simulink model "gyro_read"  (R2020a)
settings: Solver=FixedStepDiscrete  StartTime=0.0  StopTime=10.0  RelTol=1e-3  EnableMultiTasking=on
undefined symbols (not defined in the file): ESP, IDF, IP, TCP
libraries: esp32_i2c_lib x15, simulink x5, waijung2_utilities_lib x4, esp32_device_config_lib x1
settings Model: Creator=Aimagin  LastModifiedBy=Aimagin
settings SolverCC: PositivePriorityOrder=on  AutoInsertRateTranBlk=on
settings OptimizationCC: DefaultParameterBehavior=Inlined  EnhancedBackFolding=on  PassReuseOutputArgsAs=Individual arguments  ZeroExternalMemoryAtStartup=off  ZeroInternalMemoryAtStartup=off  OptimizeBlockOrder=speed  DifferentSizesBufferReuse=on  OptimizationCustomize=off  EfficientTunableParamExpr=on
settings DebuggingCC: ParameterTunabilityLossMsg=error
settings HardwareCC: ProdBitPerPointer=32  ProdBitPerSizeT=32  ProdBitPerPtrDiffT=32  ProdLargestAtomicInteger=Long  ProdLargestAtomicFloat=Double  ProdWordSize=32  ProdHWDeviceType=Cadence Design Systems (Tensilica)->Espressif Xtensa single-/dual-core 32-bit LX6 microprocessor
settings SFSimCC: MATLABDynamicMemAlloc=off
settings RTWCC: Description=Waijung 2 ESP32 target  SystemTargetFile=esp32.tlc  TemplateMakefile=esp32.tmf  RetainRTWFile=on
settings CodeAppCC: ForceParamTrailComments=on  IgnoreCustomStorageClasses=off  OperatorAnnotations=on  SimulinkDataObjDesc=on  SFDataObjDesc=on  InsertBlockDesc=on
settings STFCustomTargetCC: TargetLangStandard=C99 (ISO)  MultiwordLength=256  ModelReferenceCompliant=off  CombineOutputUpdateFcns=on  ERTCustomFileBanners=on  SupportContinuousTime=off  SupportNonInlinedSFcns=off  RemoveResetFunc=on  MATLABClassNameForMDSCustomization=Simulink.SoftwareTarget.ERTCustomization  SystemTargetFile=esp32.tlc
settings ERTTargetCC: TargetLangStandard=C99 (ISO)  ModelReferenceCompliant=off  ParMdlRefBuildCompliant=off  CompOptLevelCompliant=off  ConcurrentExecutionCompliant=off  ModelStepFunctionPrototypeControlCompliant=off  CPPClassGenCompliant=off  UseToolchainInfoCompliant=off  ExtModeStaticAlloc=on  ExtModeStaticAllocSize=2048  InlinedParameterPlacement=NonHierarchical  ERTSrcFileBannerTemplate=esp32_code_template.cgt  ERTHdrFileBannerTemplate=esp32_code_template.cgt  ERTDataSrcFileTemplate=esp32_code_template.cgt  ERTDataHdrFileTemplate=esp32_code_template.cgt  ERTCustomFileTemplate=esp32_file_process.tlc

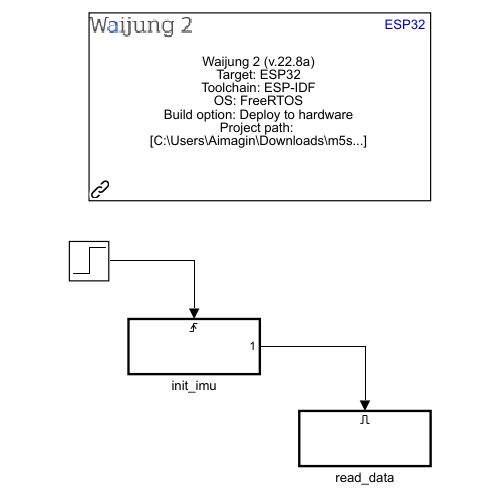
[thumbnail: Simulink's stored preview of the top-level diagram]
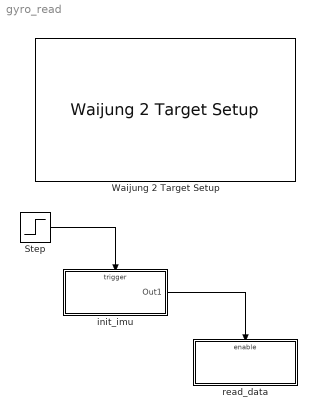
== system gyro_read ==
  Step : Step  SampleTime=0.2
  Waijung 2 Target Setup : esp32_device_config_lib/Waijung 2 Target Setup  waijungversion=22.8a  toolchain=ESP-IDF  os=FreeRTOS  sampletime=-1  simulink_managebuildsystem=on  projectpath=C:\Users\Aimagin\Downloads\m5stick_wrkshop\gyro_read_esp32_build_system  espidfpath=C:\msys32\home\skris\esp\esp-idf  buildoptions=Deploy to hardware  blockid=Waijung2TargetSetup  target=ESP32  defaultstacksize=2048  basepriority=0  highestpriority=10  generate_baserate_task=on  tickrate=1000  esp32target=ESP32  esp32targetdef=esp32  esp32flashsize=4MB  esp32comport=COM8  esp32baudrate=115200  esp32advancedconfig=off  esp32partitiontable=Use default waijung2 partition table  esp32partitionpath=Browse the partition table  partitionname=partitions.csv  editpartition=off  custompartitiondata={'nvs','data','nvs','','0x6000','';'phy_init','data','phy','','0x1000','';'factory','app','factory','','1M',''}  reqblocks=default  esp32custompartition={'nvs','data','nvs','','0x6000','';'phy_init','data','phy','','0x1000','';'factory','app','factory','','1M',''}  cominterface=TCP/IP  wifimode=WIFI AP  wifissid=esp32ssid  wifipassword=password  deviceip=192.168.1.10  targetgateway=192.168.1.1  targetnetmask=255.255.255.0  manualdns=on  targetdnsip=8.8.8.8  targetipport=256  targetipdef=0  targetmaskdef=0  targetgatewaydef=0  targetdnsipdef=0  hosttimeout=10  hostverbose=off
      settings: SourceProductName=Waijung 2 Blockset
  init_imu : Subsystem  TreatAsAtomicUnit=on
  read_data : Subsystem  TreatAsAtomicUnit=on
  wires:
  Step/1 -> init_imu/Trigger
  init_imu/1(Out1) -> read_data/Enable

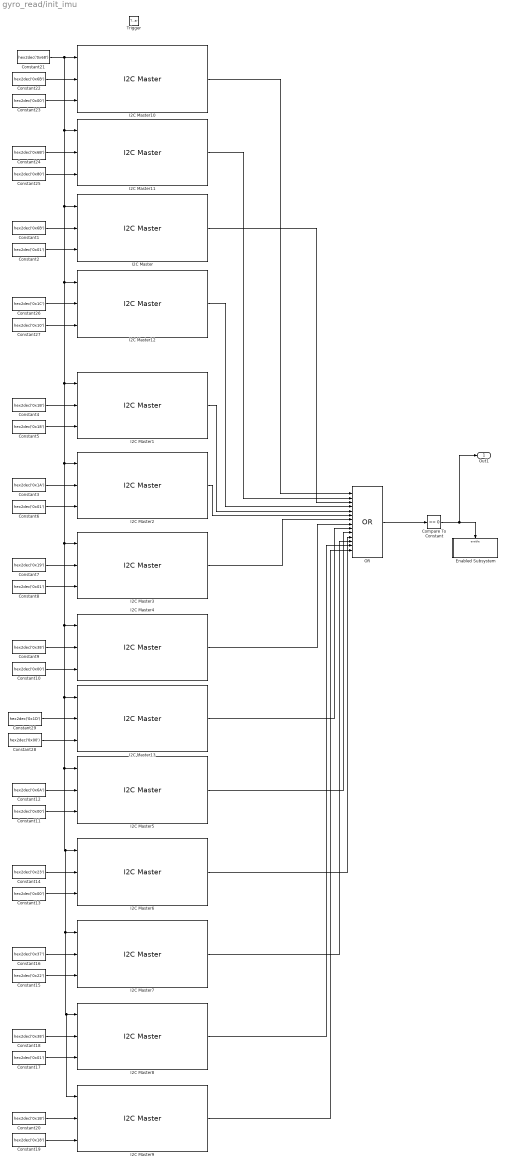
== system gyro_read/init_imu ==
  Trigger : TriggerPort  VariantControl=Variant
  Compare To Constant : simulink/Logic and Bit Operations/Compare To Constant  relop===  const=0  OutDataTypeStr=boolean
  Constant1 : Constant  Value=hex2dec('0x6B')  SampleTime=-1
  Constant{10..11,13,23,28} (5 alike) : Constant  Value=hex2dec('0x00')  SampleTime=-1
  Constant12 : Constant  Value=hex2dec('0x6A')  SampleTime=-1
  Constant14 : Constant  Value=hex2dec('0x23')  SampleTime=-1
  Constant15 : Constant  Value=hex2dec('0x22')  SampleTime=-1
  Constant16 : Constant  Value=hex2dec('0x37')  SampleTime=-1
  Constant{2,6,8,17} (4 alike) : Constant  Value=hex2dec('0x01')  SampleTime=-1
  Constant18 : Constant  Value=hex2dec('0x38')  SampleTime=-1
  Constant19 : Constant  Value=hex2dec('0x18')  SampleTime=-1
  Constant20 : Constant  Value=hex2dec('0x1B')  SampleTime=-1
  Constant21 : Constant  Value=hex2dec('0x68')  SampleTime=-1
  Constant22 : Constant  Value=hex2dec('0x6B')  SampleTime=-1
  Constant24 : Constant  Value=hex2dec('0x6B')  SampleTime=-1
  Constant25 : Constant  Value=hex2dec('0x80')  SampleTime=-1
  Constant26 : Constant  Value=hex2dec('0x1C')  SampleTime=-1
  Constant27 : Constant  Value=hex2dec('0x10')  SampleTime=-1
  Constant29 : Constant  Value=hex2dec('0x1D')  SampleTime=-1
  Constant3 : Constant  Value=hex2dec('0x1A')  SampleTime=-1
  Constant4 : Constant  Value=hex2dec('0x1B')  SampleTime=-1
  Constant5 : Constant  Value=hex2dec('0x18')  SampleTime=-1
  Constant7 : Constant  Value=hex2dec('0x19')  SampleTime=-1
  Constant9 : Constant  Value=hex2dec('0x38')  SampleTime=-1
  Enabled Subsystem : Subsystem  TreatAsAtomicUnit=on
  I2C Master : esp32_i2c_lib/I2C Master  blockid=init_imuI2CMaster  mode=Continuous  i2cinit=on  i2cport=0  i2cportdef=I2C_NUM_0  clkspeed=100  overridepin=off  sdapin=21  sdapinpull=Enable  sclpin=22  sclpinpull=Enable  inputcount=2  outputcount=0  enablelog=off  inputportlabel={'SlvAddr' 'Wr0 (uint8)' 'Wr1 (uint8)' }  outputportlabel={'Status' '(uint8) Rd0' '(uint8) Rd1' }  sdapinpulldef=GPIO_PULLUP_ENABLE  sclpinpulldef=GPIO_PULLUP_ENABLE  enablelogdef=0  sampletime=-1  sampletimestr=2
      settings: SourceProductName=Waijung 2 Blockset
  I2C Master1 : esp32_i2c_lib/I2C Master  blockid=init_imuI2CMaster1  mode=Continuous  i2cinit=off  i2cport=0  i2cportdef=I2C_NUM_0  clkspeed=100  overridepin=off  sdapin=21  sdapinpull=Enable  sclpin=22  sclpinpull=Enable  inputcount=2  outputcount=0  enablelog=off  inputportlabel={'SlvAddr' 'Wr0 (uint8)' 'Wr1 (uint8)' }  outputportlabel={'Status' '(uint8) Rd0' '(uint8) Rd1' }  sdapinpulldef=GPIO_PULLUP_ENABLE  sclpinpulldef=GPIO_PULLUP_ENABLE  enablelogdef=0  sampletime=-1  sampletimestr=2
      settings: SourceProductName=Waijung 2 Blockset
  I2C Master10 : esp32_i2c_lib/I2C Master  blockid=init_imuI2CMaster10  mode=Continuous  i2cinit=off  i2cport=0  i2cportdef=I2C_NUM_0  clkspeed=100  overridepin=off  sdapin=21  sdapinpull=Enable  sclpin=22  sclpinpull=Enable  inputcount=2  outputcount=0  enablelog=off  inputportlabel={'SlvAddr' 'Wr0 (uint8)' 'Wr1 (uint8)' }  outputportlabel={'Status' '(uint8) Rd0' '(uint8) Rd1' }  sdapinpulldef=GPIO_PULLUP_ENABLE  sclpinpulldef=GPIO_PULLUP_ENABLE  enablelogdef=0  sampletime=-1  sampletimestr=2
      settings: SourceProductName=Waijung 2 Blockset
  I2C Master11 : esp32_i2c_lib/I2C Master  blockid=init_imuI2CMaster11  mode=Continuous  i2cinit=off  i2cport=0  i2cportdef=I2C_NUM_0  clkspeed=100  overridepin=off  sdapin=21  sdapinpull=Enable  sclpin=22  sclpinpull=Enable  inputcount=2  outputcount=0  enablelog=off  inputportlabel={'SlvAddr' 'Wr0 (uint8)' 'Wr1 (uint8)' }  outputportlabel={'Status' '(uint8) Rd0' '(uint8) Rd1' }  sdapinpulldef=GPIO_PULLUP_ENABLE  sclpinpulldef=GPIO_PULLUP_ENABLE  enablelogdef=0  sampletime=-1  sampletimestr=2
      settings: SourceProductName=Waijung 2 Blockset
  I2C Master12 : esp32_i2c_lib/I2C Master  blockid=init_imuI2CMaster12  mode=Continuous  i2cinit=off  i2cport=0  i2cportdef=I2C_NUM_0  clkspeed=100  overridepin=off  sdapin=21  sdapinpull=Enable  sclpin=22  sclpinpull=Enable  inputcount=2  outputcount=0  enablelog=off  inputportlabel={'SlvAddr' 'Wr0 (uint8)' 'Wr1 (uint8)' }  outputportlabel={'Status' '(uint8) Rd0' '(uint8) Rd1' }  sdapinpulldef=GPIO_PULLUP_ENABLE  sclpinpulldef=GPIO_PULLUP_ENABLE  enablelogdef=0  sampletime=-1  sampletimestr=2
      settings: SourceProductName=Waijung 2 Blockset
  I2C Master13 : esp32_i2c_lib/I2C Master  blockid=init_imuI2CMaster13  mode=Continuous  i2cinit=off  i2cport=0  i2cportdef=I2C_NUM_0  clkspeed=100  overridepin=off  sdapin=21  sdapinpull=Enable  sclpin=22  sclpinpull=Enable  inputcount=2  outputcount=0  enablelog=off  inputportlabel={'SlvAddr' 'Wr0 (uint8)' 'Wr1 (uint8)' }  outputportlabel={'Status' '(uint8) Rd0' '(uint8) Rd1' }  sdapinpulldef=GPIO_PULLUP_ENABLE  sclpinpulldef=GPIO_PULLUP_ENABLE  enablelogdef=0  sampletime=-1  sampletimestr=2
      settings: SourceProductName=Waijung 2 Blockset
  I2C Master2 : esp32_i2c_lib/I2C Master  blockid=init_imuI2CMaster2  mode=Continuous  i2cinit=off  i2cport=0  i2cportdef=I2C_NUM_0  clkspeed=100  overridepin=off  sdapin=21  sdapinpull=Enable  sclpin=22  sclpinpull=Enable  inputcount=2  outputcount=0  enablelog=off  inputportlabel={'SlvAddr' 'Wr0 (uint8)' 'Wr1 (uint8)' }  outputportlabel={'Status' '(uint8) Rd0' '(uint8) Rd1' }  sdapinpulldef=GPIO_PULLUP_ENABLE  sclpinpulldef=GPIO_PULLUP_ENABLE  enablelogdef=0  sampletime=-1  sampletimestr=2
      settings: SourceProductName=Waijung 2 Blockset
  I2C Master3 : esp32_i2c_lib/I2C Master  blockid=init_imuI2CMaster3  mode=Continuous  i2cinit=off  i2cport=0  i2cportdef=I2C_NUM_0  clkspeed=100  overridepin=off  sdapin=21  sdapinpull=Enable  sclpin=22  sclpinpull=Enable  inputcount=2  outputcount=0  enablelog=off  inputportlabel={'SlvAddr' 'Wr0 (uint8)' 'Wr1 (uint8)' }  outputportlabel={'Status' '(uint8) Rd0' '(uint8) Rd1' }  sdapinpulldef=GPIO_PULLUP_ENABLE  sclpinpulldef=GPIO_PULLUP_ENABLE  enablelogdef=0  sampletime=-1  sampletimestr=2
      settings: SourceProductName=Waijung 2 Blockset
  I2C Master4 : esp32_i2c_lib/I2C Master  blockid=init_imuI2CMaster4  mode=Continuous  i2cinit=off  i2cport=0  i2cportdef=I2C_NUM_0  clkspeed=100  overridepin=off  sdapin=21  sdapinpull=Enable  sclpin=22  sclpinpull=Enable  inputcount=2  outputcount=0  enablelog=off  inputportlabel={'SlvAddr' 'Wr0 (uint8)' 'Wr1 (uint8)' }  outputportlabel={'Status' '(uint8) Rd0' '(uint8) Rd1' }  sdapinpulldef=GPIO_PULLUP_ENABLE  sclpinpulldef=GPIO_PULLUP_ENABLE  enablelogdef=0  sampletime=-1  sampletimestr=2
      settings: SourceProductName=Waijung 2 Blockset
  I2C Master5 : esp32_i2c_lib/I2C Master  blockid=init_imuI2CMaster5  mode=Continuous  i2cinit=off  i2cport=0  i2cportdef=I2C_NUM_0  clkspeed=100  overridepin=off  sdapin=21  sdapinpull=Enable  sclpin=22  sclpinpull=Enable  inputcount=2  outputcount=0  enablelog=off  inputportlabel={'SlvAddr' 'Wr0 (uint8)' 'Wr1 (uint8)' }  outputportlabel={'Status' '(uint8) Rd0' '(uint8) Rd1' }  sdapinpulldef=GPIO_PULLUP_ENABLE  sclpinpulldef=GPIO_PULLUP_ENABLE  enablelogdef=0  sampletime=-1  sampletimestr=2
      settings: SourceProductName=Waijung 2 Blockset
  I2C Master6 : esp32_i2c_lib/I2C Master  blockid=init_imuI2CMaster6  mode=Continuous  i2cinit=off  i2cport=0  i2cportdef=I2C_NUM_0  clkspeed=100  overridepin=off  sdapin=21  sdapinpull=Enable  sclpin=22  sclpinpull=Enable  inputcount=2  outputcount=0  enablelog=off  inputportlabel={'SlvAddr' 'Wr0 (uint8)' 'Wr1 (uint8)' }  outputportlabel={'Status' '(uint8) Rd0' '(uint8) Rd1' }  sdapinpulldef=GPIO_PULLUP_ENABLE  sclpinpulldef=GPIO_PULLUP_ENABLE  enablelogdef=0  sampletime=-1  sampletimestr=2
      settings: SourceProductName=Waijung 2 Blockset
  I2C Master7 : esp32_i2c_lib/I2C Master  blockid=init_imuI2CMaster7  mode=Continuous  i2cinit=off  i2cport=0  i2cportdef=I2C_NUM_0  clkspeed=100  overridepin=off  sdapin=21  sdapinpull=Enable  sclpin=22  sclpinpull=Enable  inputcount=2  outputcount=0  enablelog=off  inputportlabel={'SlvAddr' 'Wr0 (uint8)' 'Wr1 (uint8)' }  outputportlabel={'Status' '(uint8) Rd0' '(uint8) Rd1' }  sdapinpulldef=GPIO_PULLUP_ENABLE  sclpinpulldef=GPIO_PULLUP_ENABLE  enablelogdef=0  sampletime=-1  sampletimestr=2
      settings: SourceProductName=Waijung 2 Blockset
  I2C Master8 : esp32_i2c_lib/I2C Master  blockid=init_imuI2CMaster8  mode=Continuous  i2cinit=off  i2cport=0  i2cportdef=I2C_NUM_0  clkspeed=100  overridepin=off  sdapin=21  sdapinpull=Enable  sclpin=22  sclpinpull=Enable  inputcount=2  outputcount=0  enablelog=off  inputportlabel={'SlvAddr' 'Wr0 (uint8)' 'Wr1 (uint8)' }  outputportlabel={'Status' '(uint8) Rd0' '(uint8) Rd1' }  sdapinpulldef=GPIO_PULLUP_ENABLE  sclpinpulldef=GPIO_PULLUP_ENABLE  enablelogdef=0  sampletime=-1  sampletimestr=2
      settings: SourceProductName=Waijung 2 Blockset
  I2C Master9 : esp32_i2c_lib/I2C Master  blockid=init_imuI2CMaster9  mode=Continuous  i2cinit=off  i2cport=0  i2cportdef=I2C_NUM_0  clkspeed=100  overridepin=off  sdapin=21  sdapinpull=Enable  sclpin=22  sclpinpull=Enable  inputcount=2  outputcount=0  enablelog=off  inputportlabel={'SlvAddr' 'Wr0 (uint8)' 'Wr1 (uint8)' }  outputportlabel={'Status' '(uint8) Rd0' '(uint8) Rd1' }  sdapinpulldef=GPIO_PULLUP_ENABLE  sclpinpulldef=GPIO_PULLUP_ENABLE  enablelogdef=0  sampletime=-1  sampletimestr=2
      settings: SourceProductName=Waijung 2 Blockset
  OR : Logic  Operator=OR  Inputs=14  IconShape=distinctive  AllPortsSameDT=off  OutDataTypeStr=boolean
  Out1 : Outport
  wires:
  Constant1/1 -> I2C Master/2
  Constant2/1 -> I2C Master/3
  Constant5/1 -> I2C Master1/3
  Constant4/1 -> I2C Master1/2
  Constant3/1 -> I2C Master2/2
  Constant6/1 -> I2C Master2/3
  Constant8/1 -> I2C Master3/3
  Constant7/1 -> I2C Master3/2
  Constant9/1 -> I2C Master4/2
  Constant10/1 -> I2C Master4/3
  Constant11/1 -> I2C Master5/3
  Constant12/1 -> I2C Master5/2
  Constant14/1 -> I2C Master6/2
  Constant13/1 -> I2C Master6/3
  Constant15/1 -> I2C Master7/3
  Constant16/1 -> I2C Master7/2
  Constant18/1 -> I2C Master8/2
  Constant17/1 -> I2C Master8/3
  Constant19/1 -> I2C Master9/3
  Constant20/1 -> I2C Master9/2
  Constant21/1 -> I2C Master11/1, I2C Master12/1, I2C Master13/1, I2C Master9/1, I2C Master8/1, I2C Master7/1, I2C Master6/1, I2C Master5/1, I2C Master4/1, I2C Master3/1, I2C Master2/1, I2C Master1/1, I2C Master/1, I2C Master10/1
  Compare To Constant/1 -> Out1/1, Enabled Subsystem/Enable
  OR/1 -> Compare To Constant/1
  Constant23/1 -> I2C Master10/3
  Constant22/1 -> I2C Master10/2
  Constant24/1 -> I2C Master11/2
  Constant25/1 -> I2C Master11/3
  Constant26/1 -> I2C Master12/2
  Constant27/1 -> I2C Master12/3
  Constant29/1 -> I2C Master13/2
  Constant28/1 -> I2C Master13/3
  I2C Master10/1 -> OR/1
  I2C Master11/1 -> OR/2
  I2C Master/1 -> OR/3
  I2C Master12/1 -> OR/4
  I2C Master1/1 -> OR/5
  I2C Master2/1 -> OR/6
  I2C Master3/1 -> OR/7
  I2C Master4/1 -> OR/8
  I2C Master13/1 -> OR/9
  I2C Master5/1 -> OR/10
  I2C Master6/1 -> OR/11
  I2C Master7/1 -> OR/12
  I2C Master8/1 -> OR/13
  I2C Master9/1 -> OR/14

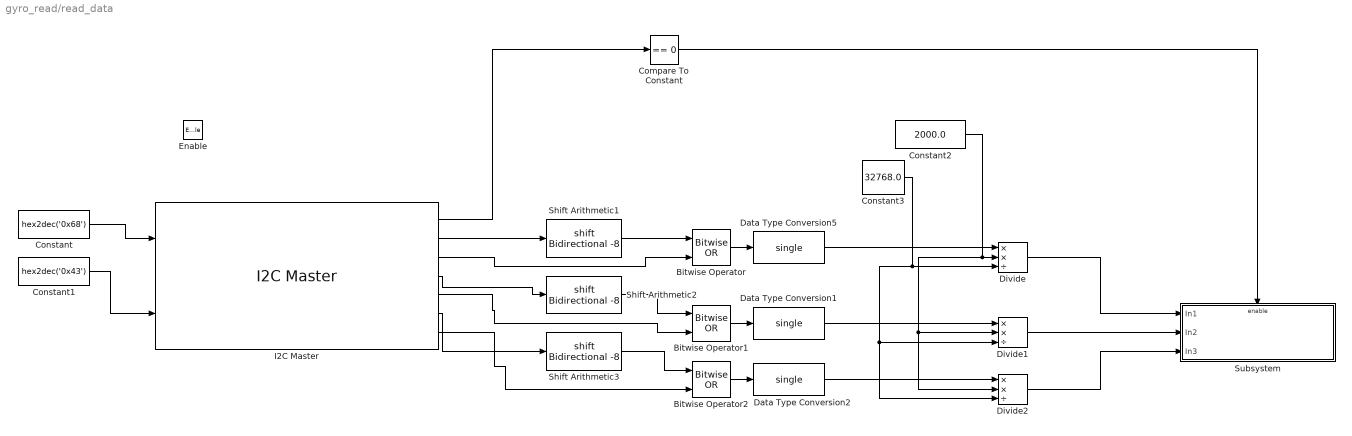
== system gyro_read/read_data ==
  Enable : EnablePort
  Bitwise Operator : simulink/Logic and Bit Operations/Bitwise Operator  logicop=OR  UseBitMask=off  NumInputPorts=2  BitMask=bin2dec('11011001')  BitMaskRealWorld=Stored Integer
  Bitwise Operator1 : simulink/Logic and Bit Operations/Bitwise Operator  logicop=OR  UseBitMask=off  NumInputPorts=2  BitMask=bin2dec('11011001')  BitMaskRealWorld=Stored Integer
  Bitwise Operator2 : simulink/Logic and Bit Operations/Bitwise Operator  logicop=OR  UseBitMask=off  NumInputPorts=2  BitMask=bin2dec('11011001')  BitMaskRealWorld=Stored Integer
  Compare To Constant : simulink/Logic and Bit Operations/Compare To Constant  relop===  const=0  OutDataTypeStr=boolean
  Constant : Constant  Value=hex2dec('0x68')  SampleTime=-1
  Constant1 : Constant  Value=hex2dec('0x43')  SampleTime=-1
  Constant2 : Constant  Value=2000.0  SampleTime=-1
  Constant3 : Constant  Value=32768.0  SampleTime=-1
  Data Type Conversion1 : DataTypeConversion  OutDataTypeStr=single
  Data Type Conversion2 : DataTypeConversion  OutDataTypeStr=single
  Data Type Conversion5 : DataTypeConversion  OutDataTypeStr=single
  Divide : Product  Inputs=**/
  Divide1 : Product  Inputs=**/
  Divide2 : Product  Inputs=**/
  I2C Master : esp32_i2c_lib/I2C Master  blockid=read_dataI2CMaster  mode=Continuous  i2cinit=off  i2cport=0  i2cportdef=I2C_NUM_0  clkspeed=100  overridepin=off  sdapin=21  sdapinpull=Enable  sclpin=22  sclpinpull=Enable  inputcount=1  outputcount=6  enablelog=off  inputportlabel={'SlvAddr' 'Wr0 (uint8)' 'Wr1 (uint8)' }  outputportlabel={'Status' '(uint8) Rd0' '(uint8) Rd1' }  sdapinpulldef=GPIO_PULLUP_ENABLE  sclpinpulldef=GPIO_PULLUP_ENABLE  enablelogdef=0  sampletime=-1  sampletimestr=2
      settings: SourceProductName=Waijung 2 Blockset
  Shift Arithmetic1 : ArithShift  BitShiftNumber=-8
  Shift Arithmetic2 : ArithShift  BitShiftNumber=-8
  Shift Arithmetic3 : ArithShift  BitShiftNumber=-8
  Subsystem : Subsystem
  wires:
  Constant1/1 -> I2C Master/2
  Constant/1 -> I2C Master/1
  I2C Master/2 -> Shift Arithmetic1/1
  Shift Arithmetic1/1 -> Bitwise Operator/1
  I2C Master/3 -> Bitwise Operator/2
  Bitwise Operator/1 -> Data Type Conversion5/1
  Bitwise Operator1/1 -> Data Type Conversion1/1
  I2C Master/5 -> Bitwise Operator1/2
  Shift Arithmetic2/1 -> Bitwise Operator1/1
  I2C Master/4 -> Shift Arithmetic2/1
  I2C Master/6 -> Shift Arithmetic3/1
  Shift Arithmetic3/1 -> Bitwise Operator2/1
  I2C Master/7 -> Bitwise Operator2/2
  Bitwise Operator2/1 -> Data Type Conversion2/1
  Data Type Conversion5/1 -> Divide/1
  Constant2/1 -> Divide2/2, Divide1/2, Divide/2
  Constant3/1 -> Divide2/3, Divide1/3, Divide/3
  Data Type Conversion1/1 -> Divide1/1
  Data Type Conversion2/1 -> Divide2/1
  Divide/1 -> Subsystem/1(In1)
  Divide1/1 -> Subsystem/2(In2)
  Divide2/1 -> Subsystem/3(In3)
  I2C Master/1 -> Compare To Constant/1
  Compare To Constant/1 -> Subsystem/Enable

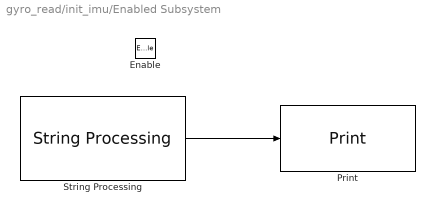
== system gyro_read/init_imu/Enabled Subsystem ==
  Enable : EnablePort
  Print : waijung2_utilities_lib/Print  printfcn=printf  strinput=Character Vector  sampletime=-1  blockid=init_imuEnabledSubsystemPrint  sampletimestr=2
      settings: SourceProductName=Waijung 2 Blockset
  String Processing : waijung2_utilities_lib/String Processing  conf=processing  stringfunction=sprintf  stringformat='Successfully initialize the IMU\n'  begindelimiter=''  enddelimiter=''  buffersize=64  enablestatus=off  use_pointer=off  pointer_list="\"\""  string_pointer=off  portpinstr=0  sampletime=-1  blockid=init_imuEnabledSubsystemStringProcessing  inputporttype=[]  inputportwidth=[]  inputportlabel={}  outputporttype=[3]  outputportwidth=[64]  outputportlabel={'Output'}  compat=0  optionstring="[\"Param1\",\"Param1\"]"  datatypestring=[]
      settings: SourceProductName=Waijung 2 Blockset
  wires:
  String Processing/1 -> Print/1

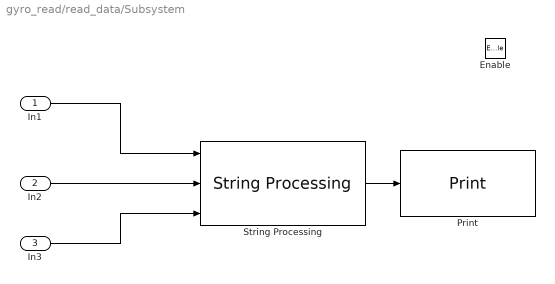
== system gyro_read/read_data/Subsystem ==
  In1 : Inport
  In2 : Inport  Port=2
  In3 : Inport  Port=3
  Enable : EnablePort
  Print : waijung2_utilities_lib/Print  printfcn=printf  strinput=Character Vector  sampletime=-1  blockid=read_dataSubsystemPrint  sampletimestr=2
      settings: SourceProductName=Waijung 2 Blockset
  String Processing : waijung2_utilities_lib/String Processing  conf=processing  stringfunction=sprintf  stringformat='gx : %f , gy : %f , gz : %f\n'  begindelimiter=''  enddelimiter=''  buffersize=128  enablestatus=off  use_pointer=off  pointer_list="\"\""  string_pointer=off  portpinstr=0  sampletime=-1  blockid=read_dataSubsystemStringProcessing  inputporttype=[-1 -1 -1]  inputportwidth=[1 1 1]  inputportlabel={'%f','%f','%f'}  outputporttype=[3]  outputportwidth=[128]  outputportlabel={'Output'}  compat=0  optionstring="[\"Param1\",\"Param1\"]"  datatypestring="[\"float\",\"float\",\"float\"]"
      settings: SourceProductName=Waijung 2 Blockset
  wires:
  In2/1 -> String Processing/2
  In1/1 -> String Processing/1
  In3/1 -> String Processing/3
  String Processing/1 -> Print/1
